simulink model "planta2"  (R2023a)
settings: Solver=VariableStepAuto  StartTime=0.0  StopTime=4000  RelTol=1e-3
values from neighbouring files (symbols this model uses):
  A1 = 0.0154    [parametros.m]    (also in variables.mat)
  A2 = 5e-5    (= 5e-05)    [parametros.m]    (also in variables.mat)
  az = 0.5    [parametros.m]    (also in variables.mat)
  g = 9.8    [parametros.m]    (also in variables.mat)
  ro = 1000    [parametros.m]    (also in variables.mat)
  st_train = 0.5    [parametros.m]    (also in variables.mat)
settings Model: Creator=empg0  LastModifiedBy=empg0

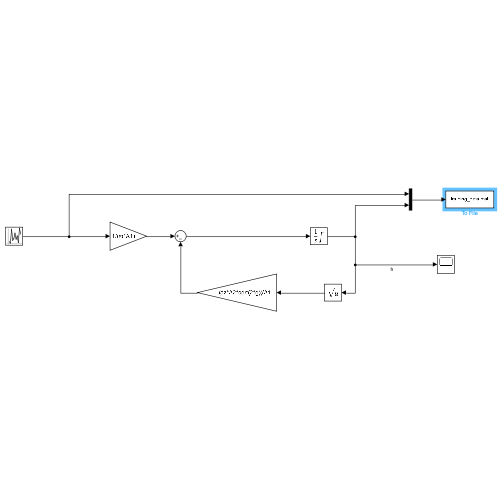
[thumbnail: Simulink's stored preview of the top-level diagram]
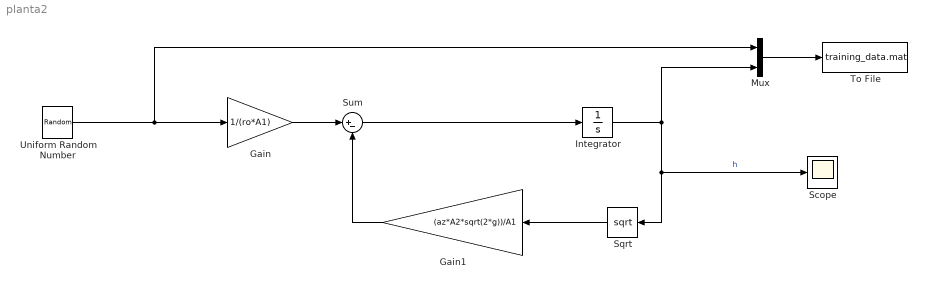
== system planta2 ==
  Gain : Gain  Gain=1/(ro*A1)
  Gain1 : Gain  Gain=(az*A2*sqrt(2*g))/A1
  Integrator : Integrator  LimitOutput=on  UpperSaturationLimit=0.62  LowerSaturationLimit=0
  Mux : Mux  Inputs=2
  Scope : Scope
  Sqrt : Sqrt
  Sum : Sum  Inputs=|+-
  To File : ToFile  Filename=training_data.mat  MatrixName=training_data  SampleTime=st_train
  Uniform Random Number : UniformRandomNumber  Minimum=0  Maximum=0.1  Seed=572  SampleTime=60
  wires:
  Uniform Random Number/1 -> Gain/1, Mux/1
  Sum/1 -> Integrator/1
  Sqrt/1 -> Gain1/1
  Gain1/1 -> Sum/2
  Gain/1 -> Sum/1
  Integrator/1 -> Mux/2, Scope/1, Sqrt/1  "h"
  Mux/1 -> To File/1
